simulink model "Trans_State2State_2020a"  (R2020a)
settings: Solver=VariableStepAuto  StartTime=0.0  StopTime=10.0  RelTol=1e-3
settings Model: Creator=apple  LastModifiedBy=apple

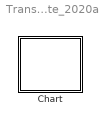
== system Trans_State2State_2020a ==
  Chart : Stateflow chart  TreatAsAtomicUnit=on

== stateflow chart Trans_State2State_2020a/Chart ==
  state On
    en:fprintf("Entry_On");
    du:fprintf("During_On");
    ex:fprintf("Exit_On");
  state Off
    en:fprintf("Entry_Off");
    du:fprintf("During_Off");
    ex:fprintf("Exit_Off");
  (default) -> On
  On -> Off : E_one/{send(E_one);}
  Off -> On : E_one
  events: E_one local RISING_EDGE_EVENT
